simulink model "Fig120"  (R2014a)
settings: Solver=FixedStepDiscrete  StartTime=0.0  StopTime=.05  FixedStep=1e-3  RelTol=1e-3
libraries: commrandsrc2 x1
settings Model: Creator=Silage  LastModifiedBy=Silage

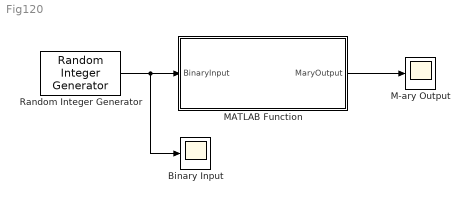
== system Fig120 ==
  Binary Input : Scope
  M-ary Output : Scope
  MATLAB Function : MATLAB Function  TreatAsAtomicUnit=on
  Random Integer Generator : commrandsrc2/Random Integer Generator  mul=2  seed=37  Ts=1e-3  frameBased=off  sampPerFrame=1  orient=off  outDataType=double
  wires:
  Random Integer Generator/1 -> Binary Input/1, MATLAB Function/1(BinaryInput)
  MATLAB Function/1(MaryOutput) -> M-ary Output/1

== matlab function Fig120/MATLAB Function ==
  data: BinaryInput input; MaryOutput output
function MaryOutput = BinaryToMary(BinaryInput)
%#codegen
persistent v1 v2 v3 vlast flag

if isempty(flag)
    flag = 1;
    v2 = 0;
    v1 = 0;
    vlast = 0;
end

v3 = v2;
v2 = v1;
v1 = BinaryInput;

if (flag == 3)
    MaryOutput = 4*v3 + 2*v2 + v1;
    vlast = MaryOutput;
    flag=1;
else
    flag = flag + 1;
    MaryOutput = vlast;
end
